simulink model "BME_333_sim1a"  (R2017a)
settings: Solver=ode4  StartTime=0.0  StopTime=20  FixedStep=.002  RelTol=1e-3
undefined symbols (not defined in the file or in its folder): B, K, M, Step
settings Model: Creator=Jake Tweedle  LastModifiedBy=Jake Tweedle

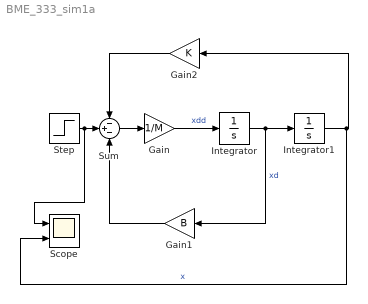
== system BME_333_sim1a ==
  Gain : Gain  Gain=1/M
  Gain1 : Gain  Gain=B
  Gain2 : Gain  Gain=K
  Integrator : Integrator
  Integrator1 : Integrator
  Scope : Scope  NumInputPorts=2
  Step : Step  Time=2  After=Step  SampleTime=0
  Sum : Sum  Inputs=-+-
  wires:
  Step/1 -> Scope/1, Sum/2
  Sum/1 -> Gain/1
  Gain/1 -> Integrator/1  "xdd"
  Integrator/1 -> Gain1/1, Integrator1/1  "xd"
  Gain1/1 -> Sum/3
  Integrator1/1 -> Scope/2, Gain2/1  "x"
  Gain2/1 -> Sum/1
